simulink model "DCmotor"  (R2023b)
settings: Solver=ode45  StartTime=0.0  StopTime=10  MaxStep=1  RelTol=1e-3  EnableMultiTasking=on
undefined symbols (not defined in the file or in its folder): Battery, Control, Environment, Motor, Vehicle
libraries: simulink x2, SignalEditorBlockLib x1
settings Model: Creator=Daniel Montesinos  LastModifiedBy=Daniel
settings SolverCC: AlgebraicLoopSolver=TrustRegion
settings DataIOCC: LimitDataPoints=on  SaveFormat=Array  SignalLoggingSaveFormat=ModelDataLogs  ReturnWorkspaceOutputs=off
settings OptimizationCC: ReuseModelBlockBuffer=off  ExpressionDepthLimit=2147483647  LifeSpan=inf
settings DebuggingCC: UnderspecifiedInitializationDetection=Classic  MergeDetectMultiDrivingBlocksExec=none  SolverPrmCheckMsg=warning  FcnCallInpInsideContextMsg=warning  UnconnectedInputMsg=warning  UnconnectedOutputMsg=warning  UnconnectedLineMsg=warning  AllowSymbolicDim=off  StateNameClashWarn=warning  SFUnexpectedBacktrackingDiag=warning  SFNoUnconditionalDefaultTransitionDiag=warning  SFExecutionAtInitializationDiag=none  ArithmeticOperatorsInVariantConditions=warning
settings HardwareCC: ProdBitPerPointer=32  ProdBitPerSizeT=32  ProdBitPerPtrDiffT=32  ProdLargestAtomicFloat=None  ProdIntDivRoundTo=Undefined  ProdEndianess=Unspecified  ProdWordSize=32  ProdHWDeviceType=32-bit Generic
settings ModelReferenceCC: EnableRefExpFcnMdlSchedulingChecks=on  PropagateSignalLabelsOutOfModel=off
settings SFSimCC: SimUseLocalCustomCode=off  CustomCodeUndefinedFunction=UseInterfaceOnly
settings RTWCC: RTWUseLocalCustomCode=off  DLArmComputeVersion=19.05
settings CodeAppCC: StateflowObjectComments=on
settings GRTTargetCC: TargetLangStandard=C89/C90 (ANSI)  CombineOutputUpdateFcns=off  GRTInterface=on
settings ConfigComp: CovMetricSettings=dw  CovSaveCumulativeToWorkspaceVar=on  CovSaveSingleToWorkspaceVar=on  CovExternalEMLEnable=off  CovSFcnEnable=off

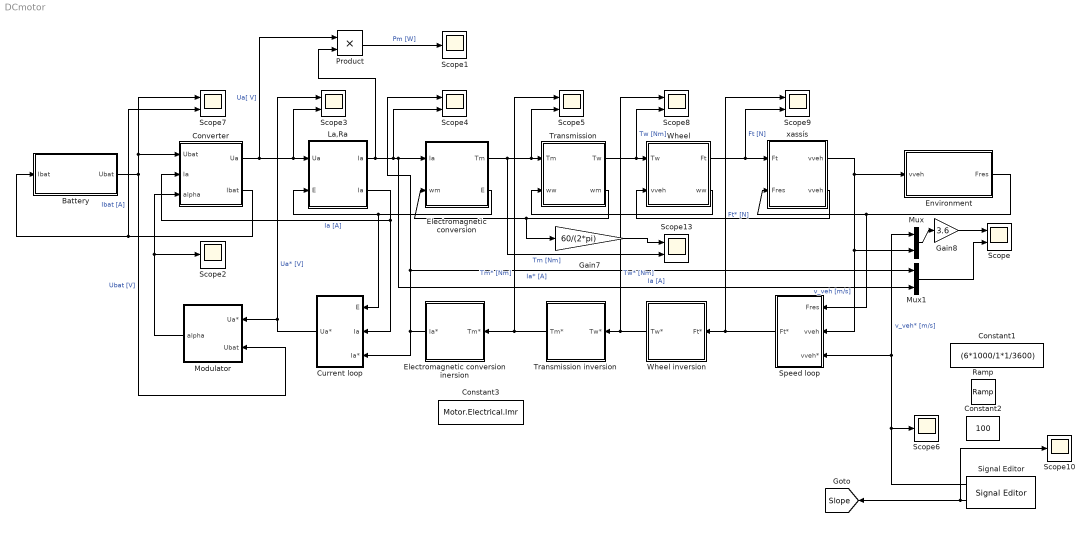
== system DCmotor ==
  Battery : Subsystem  AncestorBlock=simulink/REM/SE
      mask Display:
      | plot(0,0,100,100, 1.2*[50,57.68,60.77,63.08,64.97,66.58,68,69.26,70.4, 	71.42,72.36,78.28,80,78.28,72.36,71.42,70.4, 	69.26,68,66.58,64.97,63.08,60.77,57.68,50,42.32, 	39.23,36.92,35.03,33.42,32,30.74,29.6,28.58, 	27.64,21.72,20,21.72,27.64,28.58,29.6,30.74,32, 	33.42,35.03,36.92,39.23,42.32,50]-10, 1.2*[20,21,22,23,24,25,26,27,28,29,30,40,50,60,70,71,72, 	73,74,75,76,77,78,79,80,79,78,77,76,75,74,73,72, 	71,70,60,50,40,30,29,28,27,26,25,24,23,22,21,20]-10)
      | disp('Source')
  Constant1 : Constant  Value=(6*1000/1*1/3600)
  Constant2 : Constant  Value=100
  Constant3 : Constant  Value=Motor.Electrical.Imr
  Converter : Subsystem  AncestorBlock=simulink/REM/EC Elec  mask(Hacheur){}
      mask Display: plot(0,0,100,100,[10,10,90,90,10],[90,10,10,90,90])
  Current loop : Subsystem  AncestorBlock=simulink/SMC/Asservissement Correcteur IP
      mask Display: plot(0,0,100,100, [10,30,90,70,10,90],[90,10,10,90,90,10])
  Electromagnetic conversion : Subsystem  AncestorBlock=simulink/REM/EC EM
      mask Display: plot(0,0,100,100, 1.4*[50,57.68,60.77,63.08,64.97,66.58,68,69.26,70.4, 	71.42,72.36,78.28,80,78.28,72.36,71.42,70.4, 	69.26,68,66.58,64.97,63.08,60.77,57.68,50,42.32, 	39.23,36.92,35.03,33.42,32,30.74,29.6,28.58, 	27.64,21.72,20,21.72,27.64,28.58,29.6,30.74,32, 	33.42,35.03,36.92,39.23,42.32,50]-20, 1.4*[20,21,22,23,24,25,26,27,28,29,30,40,50,60,70,71,72, 	73,74,75,76,77,78,79,80,79,78,77,76,75,74,73,72, 	71,70,60,50,40,30,29,28,27,26,25,24,23,22,21,20]-20)
  Electromagnetic conversion inersion : Subsystem  AncestorBlock=simulink/SMC/Inversion EC avec mesure
      mask Display: plot(0,0,100,100,[10,30,90,70,10],[90,10,10,90,90])
  Environment : Subsystem  AncestorBlock=simulink/REM/SE
      mask Display:
      | plot(0,0,100,100, 1.2*[50,57.68,60.77,63.08,64.97,66.58,68,69.26,70.4, 	71.42,72.36,78.28,80,78.28,72.36,71.42,70.4, 	69.26,68,66.58,64.97,63.08,60.77,57.68,50,42.32, 	39.23,36.92,35.03,33.42,32,30.74,29.6,28.58, 	27.64,21.72,20,21.72,27.64,28.58,29.6,30.74,32, 	33.42,35.03,36.92,39.23,42.32,50]-10, 1.2*[20,21,22,23,24,25,26,27,28,29,30,40,50,60,70,71,72, 	73,74,75,76,77,78,79,80,79,78,77,76,75,74,73,72, 	71,70,60,50,40,30,29,28,27,26,25,24,23,22,21,20]-10)
      | disp('Source')
  Gain7 : Gain  Gain=60/(2*pi)
  Gain8 : Gain  Gain=3.6
  La,Ra : Subsystem  AncestorBlock=simulink/REM/EA  mask(CM){}
      mask Display: plot(0,0,100,100,[10,10,90,90,10],[90,10,10,90,90], [10,90],[10,90])
  Modulator : Subsystem  AncestorBlock=simulink/SMC/Inversion EC avec mesure
      mask Display: plot(0,0,100,100,[10,30,90,70,10],[90,10,10,90,90])
  Mux : Mux  Inputs=2
  Mux1 : Mux  Inputs=2
  Product : Product
  Ramp : simulink/Sources/Ramp  slope=(3*1000/1*1/3600)/2  start=0  InitialOutput=0
  Scope{,3..5,7..9,13} (8 alike) : Scope  NumInputPorts=2
  Scope{1..2,6,10} (4 alike) : Scope
  Signal Editor : SignalEditorBlockLib/Signal Editor  FileName=C:\Users\Daniel\OneDrive - Universitat Politècnica de Catalunya\CITCEA-UPC\CITCEA\Formació\2023_09_ANJORVE_FOC\Lab2. PMSM dq control\SpeedRef.mat  ActiveScenario=Scenario  ActiveSignal=Speed  IsBus=off  OutputBusObjectStr=Bus: BusObject  SampleTime=0  ZeroCross=off  OutputAfterFinalValue=Setting to zero  Unit=inherit  PreserveSignalName=on  ApplySigPropsToAllScenarios=on  ApplySigPropsToAllSignals=off
  Speed loop : Subsystem  AncestorBlock=simulink/SMC/Asservissement Correcteur IP
      mask Display: plot(0,0,100,100, [10,30,90,70,10,90],[90,10,10,90,90,10])
  Transmission : Subsystem  AncestorBlock=simulink/REM/EC Elec  mask(Hacheur){}
      mask Display: plot(0,0,100,100,[10,10,90,90,10],[90,10,10,90,90])
  Transmission inversion : Subsystem  AncestorBlock=simulink/SMC/Inversion EC avec mesure
      mask Display: plot(0,0,100,100,[10,30,90,70,10],[90,10,10,90,90])
  Wheel : Subsystem  AncestorBlock=simulink/REM/EC Elec  mask(Hacheur){}
      mask Display: plot(0,0,100,100,[10,10,90,90,10],[90,10,10,90,90])
  Wheel inversion : Subsystem  AncestorBlock=simulink/SMC/Inversion EC avec mesure
      mask Display: plot(0,0,100,100,[10,30,90,70,10],[90,10,10,90,90])
  xassís : Subsystem  AncestorBlock=simulink/REM/EA  mask(CM){}
      mask Display: plot(0,0,100,100,[10,10,90,90,10],[90,10,10,90,90], [10,90],[10,90])
  tag scope: Slope=global
  wires:
  xassís/1(vveh) -> Environment/1(vveh), Speed loop/2(vveh), Mux/2  "v_veh [m/s]"
  Environment/1(Fres) -> xassís/2(Fres), Speed loop/1(Fres)
  Mux/1 -> Gain8/1
  xassís/2("vveh ") -> Wheel/2(vveh)
  Transmission/1(Tw) -> Scope8/2, Wheel/1(Tw)  "Tw [Nm]"
  Wheel/2(ww) -> Transmission/2(ww)
  Wheel inversion/1(Tw*) -> Transmission inversion/1(Tw*), Scope8/1  "Tw* [Nm]"
  Transmission/2(wm) -> Gain7/1, Electromagnetic conversion/2(wm)
  Electromagnetic conversion/1(Tm) -> Scope13/2, Scope5/2, Transmission/1(Tm)  "Tm [Nm]"
  La,Ra/1("Ia ") -> Product/2, Electromagnetic conversion/1(Ia), Mux1/2, Scope4/2  "Ia [A]"
  Electromagnetic conversion/2(E) -> La,Ra/2(E), Current loop/1(E)
  Electromagnetic conversion inersion/1(Ia*) -> Current loop/3(Ia*), Scope4/1, Mux1/1  "Ia* [A]"
  La,Ra/2(Ia) -> Converter/2(Ia), Current loop/2(Ia)  "Ia [A]"
  Transmission inversion/1(Tm*) -> Electromagnetic conversion inersion/1(Tm*), Scope5/1  "Tm* [Nm]"
  Modulator/1(alpha) -> Scope2/1, Converter/3(alpha)
  Converter/2(Ibat) -> Scope7/2, Battery/1(Ibat)  "Ibat [A]"
  Battery/1(Ubat) -> Modulator/2(Ubat), Scope7/1, Converter/1(Ubat)  "Ubat [V]"
  Speed loop/1(Ft*) -> Scope9/1, Wheel inversion/1(Ft*)  "Ft* [N]"
  Wheel/1(Ft) -> Scope9/2, xassís/1(Ft)  "Ft [N]"
  Current loop/1(Ua*) -> Scope3/1, Modulator/1(Ua*)  "Ua* [V]"
  Converter/1(Ua) -> Scope3/2, La,Ra/1(Ua), Product/1  "Ua[ V]"
  Gain7/1 -> Scope13/1
  Gain8/1 -> Scope/1
  Mux1/1 -> Scope/2
  Signal Editor/1 -> Scope6/1, Mux/1, Speed loop/3(vveh*)  "v_veh* [m/s]"
  Product/1 -> Scope1/1  "Pm [W]"
  Signal Editor/2 -> Scope10/1, [Slope]

== system DCmotor/Battery ==
  Ibat : Inport
  Constant : Constant  Value=Battery.Electrical.Ubat
  Terminator : Terminator
  Ubat : Outport  InitialOutput=0  VectorParamsAs1DForOutWhenUnconnected=off
  wires:
  Ibat/1 -> Terminator/1
  Constant/1 -> Ubat/1

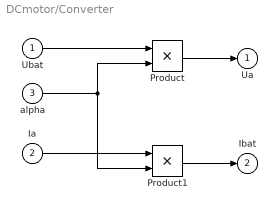
== system DCmotor/Converter ==
  Ubat : Inport
  Ia : Inport  Port=2
  alpha : Inport  Port=3
  Product : Product
  Product1 : Product
  Ua : Outport  InitialOutput=0  VectorParamsAs1DForOutWhenUnconnected=off
  Ibat : Outport  Port=2  InitialOutput=0  VectorParamsAs1DForOutWhenUnconnected=off
  wires:
  Ubat/1 -> Product/1
  alpha/1 -> Product/2, Product1/2
  Product/1 -> Ua/1
  Product1/1 -> Ibat/1
  Ia/1 -> Product1/1

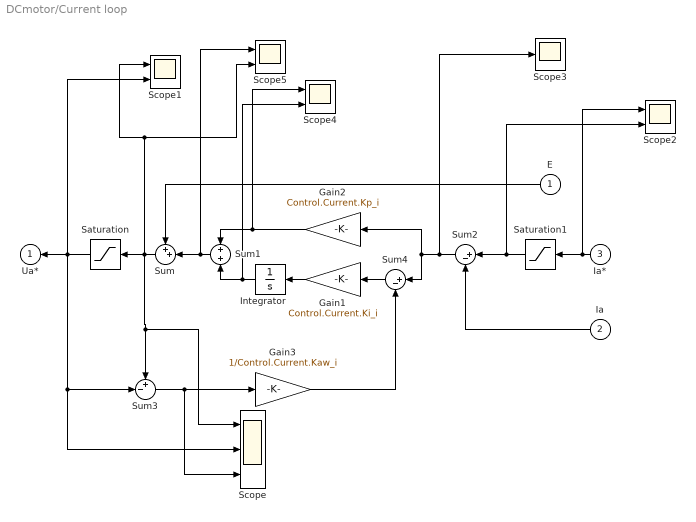
== system DCmotor/Current loop ==
  E : Inport
  Ia : Inport  Port=2
  Ia* : Inport  Port=3
  Gain1 : Gain  Gain=Control.Current.Ki_i
  Gain2 : Gain  Gain=Control.Current.Kp_i
  Gain3 : Gain  Gain=1/Control.Current.Kaw_i
  Integrator : Integrator
  Saturation : Saturate  UpperLimit=Motor.Electrical.Umr  LowerLimit=-Motor.Electrical.Umr
  Saturation1 : Saturate  UpperLimit=Motor.Electrical.Imr  LowerLimit=-Motor.Electrical.Imr
  Scope : Scope  NumInputPorts=3
  Scope{1..2,4..5} (4 alike) : Scope  NumInputPorts=2
  Scope3 : Scope
  Sum : Sum  Inputs=++|
  Sum1 : Sum
  Sum2 : Sum  Inputs=|+-
  Sum3 : Sum  Inputs=+-|
  Sum4 : Sum  Inputs=|+-
  Ua* : Outport  InitialOutput=0  VectorParamsAs1DForOutWhenUnconnected=off
  wires:
  Ia/1 -> Sum2/2
  Sum2/1 -> Scope3/1, Sum4/1, Gain2/1
  Sum1/1 -> Scope5/1, Sum/2
  Gain2/1 -> Scope4/1, Sum1/1
  Integrator/1 -> Scope4/2, Sum1/2
  Gain1/1 -> Integrator/1
  E/1 -> Sum/1
  Sum3/1 -> Scope/3, Gain3/1
  Sum4/1 -> Gain1/1
  Gain3/1 -> Sum4/2
  Ia*/1 -> Saturation1/1, Scope2/1
  Sum/1 -> Saturation/1, Scope5/2, Scope1/1, Sum3/1, Scope/1
  Saturation1/1 -> Scope2/2, Sum2/1
  Saturation/1 -> Scope1/2, Sum3/2, Scope/2, Ua*/1

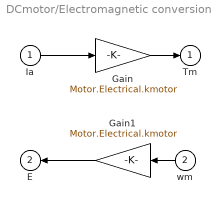
== system DCmotor/Electromagnetic conversion ==
  Ia : Inport
  wm : Inport  Port=2
  Gain : Gain  Gain=Motor.Electrical.kmotor
  Gain1 : Gain  Gain=Motor.Electrical.kmotor
  Tm : Outport  InitialOutput=0  VectorParamsAs1DForOutWhenUnconnected=off
  E : Outport  Port=2  InitialOutput=0  VectorParamsAs1DForOutWhenUnconnected=off
  wires:
  Ia/1 -> Gain/1
  Gain/1 -> Tm/1
  Gain1/1 -> E/1
  wm/1 -> Gain1/1

== system DCmotor/Electromagnetic conversion inersion ==
  Tm* : Inport
  Gain1 : Gain  Gain=1/Motor.Electrical.kmotor
  Ia* : Outport  InitialOutput=0  VectorParamsAs1DForOutWhenUnconnected=off
  wires:
  Gain1/1 -> Ia*/1
  Tm*/1 -> Gain1/1

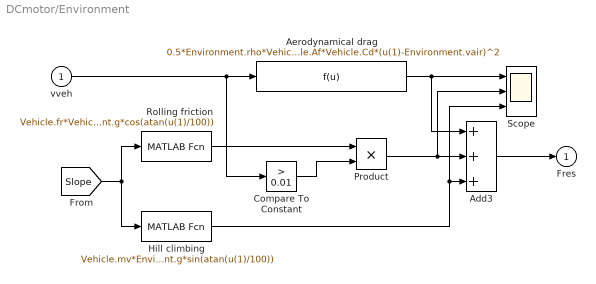
== system DCmotor/Environment ==
  vveh : Inport
  Add3 : Sum  Inputs=+++
  Aerodynamical drag : Fcn  Expr=0.5*Environment.rho*Vehicle.Af*Vehicle.Cd*(u(1)-Environment.vair)^2
  Compare To Constant : simulink/Logic and Bit Operations/Compare To Constant  relop=>  const=0.01  OutDataTypeStr=boolean  ZeroCross=off
  Hill climbing : MATLABFcn  MATLABFcn=Vehicle.mv*Environment.g*sin(atan(u(1)/100))
  Product : Product
  Rolling friction : MATLABFcn  MATLABFcn=Vehicle.fr*Vehicle.mv*Environment.g*cos(atan(u(1)/100))
  Scope : Scope  NumInputPorts=3
  Fres : Outport  InitialOutput=0  VectorParamsAs1DForOutWhenUnconnected=off
  wires:
  Aerodynamical drag/1 -> Scope/1, Add3/1
  Hill climbing/1 -> Scope/3, Add3/3
  Product/1 -> Scope/2, Add3/2
  Add3/1 -> Fres/1
  vveh/1 -> Compare To Constant/1, Aerodynamical drag/1
  Compare To Constant/1 -> Product/2
  Rolling friction/1 -> Product/1
  [Slope] -> Hill climbing/1, Rolling friction/1

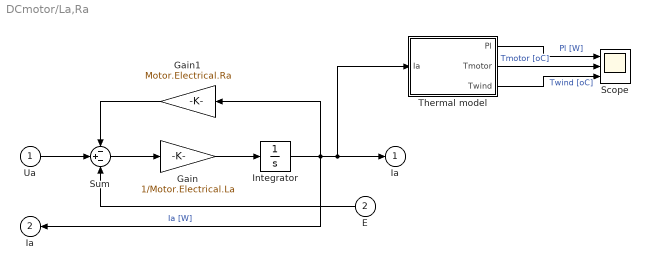
== system DCmotor/La,Ra ==
  Ua : Inport
  E : Inport  Port=2
  Gain : Gain  Gain=1/Motor.Electrical.La
  Gain1 : Gain  Gain=Motor.Electrical.Ra
  Integrator : Integrator
  Scope : Scope  NumInputPorts=3
  Sum : Sum  Inputs=-+-
  Thermal model : Subsystem
  "Ia " : Outport  InitialOutput=0  VectorParamsAs1DForOutWhenUnconnected=off
  Ia : Outport  Port=2  InitialOutput=0  VectorParamsAs1DForOutWhenUnconnected=off
  wires:
  Integrator/1 -> Ia/1, Thermal model/1(Ia), "Ia "/1, Gain1/1  "Ia [W]"
  Gain/1 -> Integrator/1
  Sum/1 -> Gain/1
  Ua/1 -> Sum/2
  Gain1/1 -> Sum/1
  E/1 -> Sum/3
  Thermal model/2(Tmotor) -> Scope/2  "Tmotor [oC]"
  Thermal model/1("Pl ") -> Scope/1  "Pl [W]"
  Thermal model/3(Twind) -> Scope/3  "Twind [oC]"

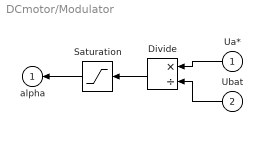
== system DCmotor/Modulator ==
  Ua* : Inport
  Ubat : Inport  Port=2
  Divide : Product  Inputs=*/
  Saturation : Saturate  UpperLimit=1  LowerLimit=-1
  alpha : Outport  InitialOutput=0  VectorParamsAs1DForOutWhenUnconnected=off
  wires:
  Divide/1 -> Saturation/1
  Ua*/1 -> Divide/1
  Ubat/1 -> Divide/2
  Saturation/1 -> alpha/1

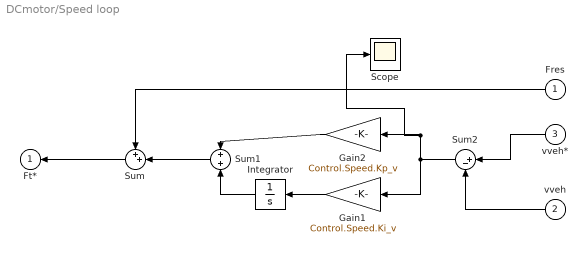
== system DCmotor/Speed loop ==
  Fres : Inport
  vveh : Inport  Port=2
  vveh* : Inport  Port=3
  Gain1 : Gain  Gain=Control.Speed.Ki_v
  Gain2 : Gain  Gain=Control.Speed.Kp_v
  Integrator : Integrator
  Scope : Scope
  Sum : Sum  Inputs=++|
  Sum1 : Sum
  Sum2 : Sum  Inputs=|+-
  Ft* : Outport  InitialOutput=0  VectorParamsAs1DForOutWhenUnconnected=off
  wires:
  Sum/1 -> Ft*/1
  Fres/1 -> Sum/1
  Gain1/1 -> Integrator/1
  Integrator/1 -> Sum1/2
  Gain2/1 -> Sum1/1
  Sum1/1 -> Sum/2
  vveh*/1 -> Sum2/1
  vveh/1 -> Sum2/2
  Sum2/1 -> Scope/1, Gain2/1, Gain1/1

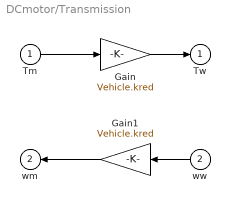
== system DCmotor/Transmission ==
  Tm : Inport
  ww : Inport  Port=2
  Gain : Gain  Gain=Vehicle.kred
  Gain1 : Gain  Gain=Vehicle.kred
  Tw : Outport  InitialOutput=0  VectorParamsAs1DForOutWhenUnconnected=off
  wm : Outport  Port=2  InitialOutput=0  VectorParamsAs1DForOutWhenUnconnected=off
  wires:
  Tm/1 -> Gain/1
  Gain/1 -> Tw/1
  Gain1/1 -> wm/1
  ww/1 -> Gain1/1

== system DCmotor/Transmission inversion ==
  Tw* : Inport
  Gain : Gain  Gain=1/Vehicle.kred
  Tm* : Outport  InitialOutput=0  VectorParamsAs1DForOutWhenUnconnected=off
  wires:
  Tw*/1 -> Gain/1
  Gain/1 -> Tm*/1

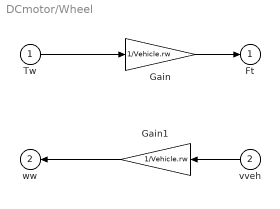
== system DCmotor/Wheel ==
  Tw : Inport
  vveh : Inport  Port=2
  Gain : Gain  Gain=1/Vehicle.rw
  Gain1 : Gain  Gain=1/Vehicle.rw
  Ft : Outport  InitialOutput=0  VectorParamsAs1DForOutWhenUnconnected=off
  ww : Outport  Port=2  InitialOutput=0  VectorParamsAs1DForOutWhenUnconnected=off
  wires:
  Tw/1 -> Gain/1
  Gain/1 -> Ft/1
  Gain1/1 -> ww/1
  vveh/1 -> Gain1/1

== system DCmotor/Wheel inversion ==
  Ft* : Inport
  Gain : Gain  Gain=Vehicle.rw
  Tw* : Outport  InitialOutput=0  VectorParamsAs1DForOutWhenUnconnected=off
  wires:
  Gain/1 -> Tw*/1
  Ft*/1 -> Gain/1

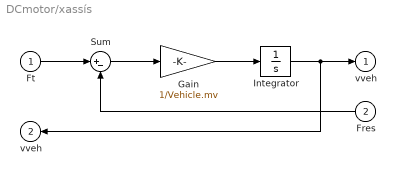
== system DCmotor/xassís ==
  Ft : Inport
  Fres : Inport  Port=2
  Gain : Gain  Gain=1/Vehicle.mv
  Integrator : Integrator
  Sum : Sum  Inputs=|+-
  vveh : Outport  InitialOutput=0  VectorParamsAs1DForOutWhenUnconnected=off
  "vveh " : Outport  Port=2  InitialOutput=0  VectorParamsAs1DForOutWhenUnconnected=off
  wires:
  Ft/1 -> Sum/1
  Fres/1 -> Sum/2
  Sum/1 -> Gain/1
  Gain/1 -> Integrator/1
  Integrator/1 -> vveh/1, "vveh "/1

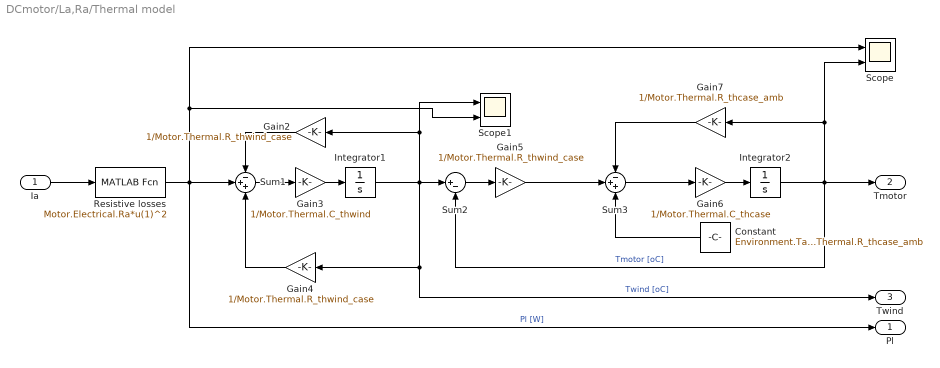
== system DCmotor/La,Ra/Thermal model ==
  Ia : Inport
  Constant : Constant  Value=Environment.Tamb/Motor.Thermal.R_thcase_amb
  Gain2 : Gain  Gain=1/Motor.Thermal.R_thwind_case
  Gain3 : Gain  Gain=1/Motor.Thermal.C_thwind
  Gain4 : Gain  Gain=1/Motor.Thermal.R_thwind_case
  Gain5 : Gain  Gain=1/Motor.Thermal.R_thwind_case
  Gain6 : Gain  Gain=1/Motor.Thermal.C_thcase
  Gain7 : Gain  Gain=1/Motor.Thermal.R_thcase_amb
  Integrator1 : Integrator
  Integrator2 : Integrator
  Resistive losses : MATLABFcn  MATLABFcn=Motor.Electrical.Ra*u(1)^2
  Scope : Scope  NumInputPorts=2
  Scope1 : Scope  NumInputPorts=2
  Sum1 : Sum  Inputs=-++
  Sum2 : Sum  Inputs=|+-
  Sum3 : Sum  Inputs=-++
  "Pl " : Outport
  Tmotor : Outport  Port=2
  Twind : Outport  Port=3
  wires:
  Gain4/1 -> Sum1/3
  Sum1/1 -> Gain3/1
  Sum2/1 -> Gain5/1
  Integrator1/1 -> Twind/1, Gain4/1, Sum2/1, Scope1/1, Gain2/1  "Twind [oC]"
  Gain6/1 -> Integrator2/1
  Integrator2/1 -> Sum2/2, Tmotor/1, Scope/2, Gain7/1  "Tmotor [oC]"
  Gain2/1 -> Sum1/1
  Sum3/1 -> Gain6/1
  Ia/1 -> Resistive losses/1
  Resistive losses/1 -> "Pl "/1, Sum1/2, Scope1/2, Scope/1  "Pl [W]"
  Gain3/1 -> Integrator1/1
  Gain7/1 -> Sum3/1
  Gain5/1 -> Sum3/2
  Constant/1 -> Sum3/3
